simulink model "privod"  (R2013a)
settings: Solver=ode45  SolverMode=SingleTasking  StartTime=0.0  StopTime=20  RelTol=1e-3  AbsTol=1e-6
settings Model: Creator=Ignatiev3  LastModifiedBy=Ignatiev3
settings SolverCC: MaxConsecutiveZCs=50000
settings DataIOCC: LimitDataPoints=off  SignalLoggingSaveFormat=ModelDataLogs
settings OptimizationCC: BlockReduction=off  BooleanDataType=off
settings DebuggingCC: SaveWithParameterizedLinksMsg=none  SignalResolutionControl=TryResolveAllWithWarning  SolverPrmCheckMsg=none  MultiTaskDSMMsg=warning  MultiTaskCondExecSysMsg=none  StrictBusMsg=None
settings HardwareCC: TargetUnknown=on
settings RTWCC: TemplateMakefile=grt_vc.tmf  IncludeERTFirstTime=on
settings GRTTargetCC: CombineOutputUpdateFcns=off  GRTInterface=on

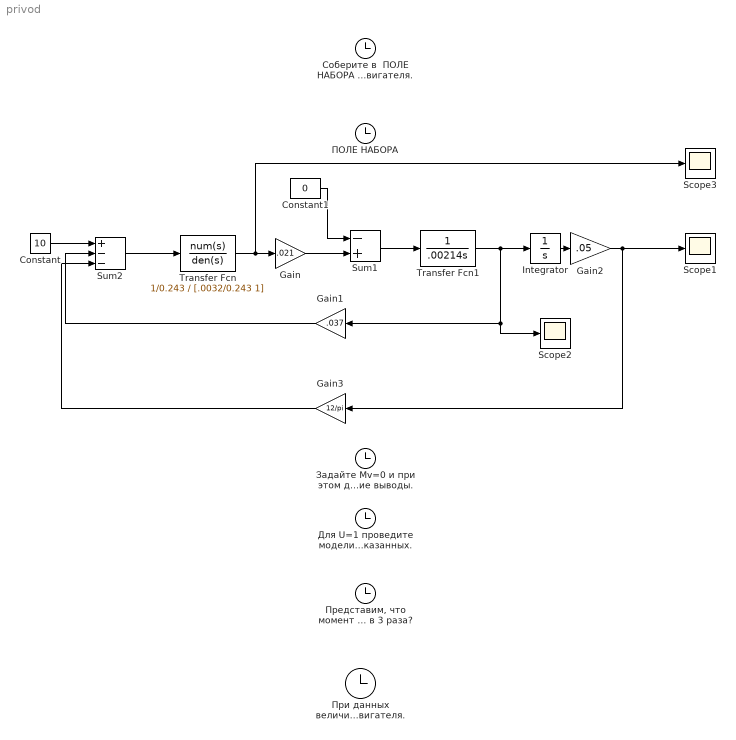
== system privod ==
  Constant : Constant  Value=10
  Constant1 : Constant  Value=0
  Gain : Gain  Gain=.021  SaturateOnIntegerOverflow=on  OutDataTypeStr=Inherit: Same as input  ParamDataTypeStr=Inherit: Same as input
  Gain1 : Gain  Gain=.037  SaturateOnIntegerOverflow=on  OutDataTypeStr=Inherit: Same as input  ParamDataTypeStr=Inherit: Same as input
  Gain2 : Gain  Gain=.05  SaturateOnIntegerOverflow=on  OutDataTypeStr=Inherit: Same as input  ParamDataTypeStr=Inherit: Same as input
  Gain3 : Gain  Gain=12/pi  SaturateOnIntegerOverflow=on  OutDataTypeStr=Inherit: Same as input  ParamDataTypeStr=Inherit: Same as input
  Integrator : Integrator
  Scope1 : Scope
      settings: TickLabels=on  YMin=3.14158  YMax=3.1416
  Scope2 : Scope
      settings: TickLabels=on  YMax=50
  Scope3 : Scope
      settings: TickLabels=on  YMax=50  SaveName=ScopeData2
  Sum1 : Sum  Inputs=-+  SaturateOnIntegerOverflow=on  InputSameDT=on  OutDataTypeStr=Inherit: Same as first input
  Sum2 : Sum  Inputs=+--  SaturateOnIntegerOverflow=on  InputSameDT=on  OutDataTypeStr=Inherit: Same as first input
  Transfer Fcn : TransferFcn  Numerator=1/0.243  Denominator=[.0032/0.243 1]
  Transfer Fcn1 : TransferFcn  Denominator=[.00214 0]
  "Для U=1 проведите моделирование переходного процесса по скорости вала двигателя для значений J=0.05; 0.1; 0.15. Сделайте вывод о влиянии момента инерции вала на скоростные качества двигателя.  Сделайте вывод,  \"насколько\"  медленнее вращается вал двигателя при увеличении момента инерции (по осциллограммам угла поворота вала дв.). Если необходимо,дополнительно задайте значения J выше указанных." : Clock
  Задайте Mv=0 и при этом для значений U=0.5; 1.5;  2 получите и зарисуйте осциллограммы скорости и угла вала двигателя. Сделайте над- лежащие выводы. : Clock
  ПОЛЕ НАБОРА : Clock
  "Представим, что момент внешних сил пропорционален с коэффициентом к=0.005: 1) скорости вращения вала дв.; 2) углу поворота вала. Иссле- дуйте моделированием влияние таких связей на переходные процессы двигателя по скорости и повороту для U=1, J=0.03. Ответьте на вопрос: как изменятся эти процессы, если коэффициент пропорциональности  внешнего момента увеличить в 3 раза?" : Clock
  "При данных величинах напряжения на якорной обмотке U и внешнего момента Mv получите и зарисуйте в отчет осциллограммы координат тока, скорости и угла поворота вала двигателя. Затем получите аналогичные осциллограммы при значениях Mv =0 и Mv = 0.15.  Сделайте соответствующий вывод о влиянии момента внешних сил на характер переходного процесса вращения вала двигателя." : Clock
  "Соберите в  ПОЛЕ НАБОРА  вторую модель, используя следующие численные значения: U=1,  Mv=0.05, T=0.01, K=0.1, k=0.1, J=0.01. Подключите виртуальные осциллографы: 1) к выходной координате вала двигателя (углу поворота) 2) через смеситель Mux к координатам тока и скорости двигателя." : Clock
  wires:
  Transfer Fcn/1 -> Scope3/1, Gain/1
  Constant/1 -> Sum2/1
  Sum2/1 -> Transfer Fcn/1
  Gain/1 -> Sum1/2
  Sum1/1 -> Transfer Fcn1/1
  Gain1/1 -> Sum2/2
  Transfer Fcn1/1 -> Scope2/1, Gain1/1, Integrator/1
  Integrator/1 -> Gain2/1
  Gain3/1 -> Sum2/3
  Gain2/1 -> Gain3/1, Scope1/1
  Constant1/1 -> Sum1/1
